simulink library "INT_AFS_DD1ms"  (R2016b)
settings: Solver=VariableStepAuto  StartTime=0.0  StopTime=10.0  RelTol=1e-3
settings Model: Creator=liutao  LastModifiedBy=liutao

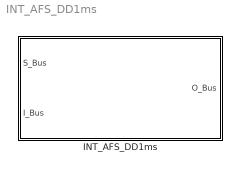
== system INT_AFS_DD1ms ==
  INT_AFS_DD1ms : Subsystem

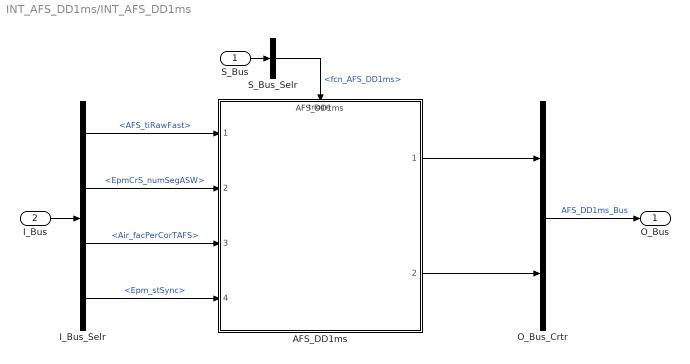
== system INT_AFS_DD1ms/INT_AFS_DD1ms ==
  S_Bus : Inport
  I_Bus : Inport  Port=2
  AFS_DD1ms : ModelReference  ModelNameDialog=AFS_DD1ms  SimulationMode=Normal  ModelReferenceVersion=1.34  TriggerPortName=function  TriggerPortTriggerType=function-call  TriggerPortStatesWhenEnabling=held
  I_Bus_Selr : BusSelector  OutputSignals=AFS_tiRawFast,EpmCrS_numSegASW,Air_facPerCorTAFS,Epm_stSync
  O_Bus_Crtr : BusCreator  Inputs=2
  S_Bus_Selr : BusSelector  OutputSignals=fcn_AFS_DD1ms
  O_Bus : Outport
  wires:
  S_Bus_Selr/1 -> AFS_DD1ms/Trigger  "<fcn_AFS_DD1ms>"
  S_Bus/1 -> S_Bus_Selr/1
  I_Bus/1 -> I_Bus_Selr/1
  I_Bus_Selr/1 -> AFS_DD1ms/1  "<AFS_tiRawFast>"
  I_Bus_Selr/2 -> AFS_DD1ms/2  "<EpmCrS_numSegASW>"
  I_Bus_Selr/3 -> AFS_DD1ms/3  "<Air_facPerCorTAFS>"
  I_Bus_Selr/4 -> AFS_DD1ms/4  "<Epm_stSync>"
  O_Bus_Crtr/1 -> O_Bus/1  "AFS_DD1ms_Bus"
  AFS_DD1ms/1 -> O_Bus_Crtr/1
  AFS_DD1ms/2 -> O_Bus_Crtr/2
